simulink model "Problem_9"  (R2020a)
settings: Solver=VariableStepAuto  StartTime=0.0  StopTime=10.0  RelTol=1e-3
settings Model: Creator=user  LastModifiedBy=user

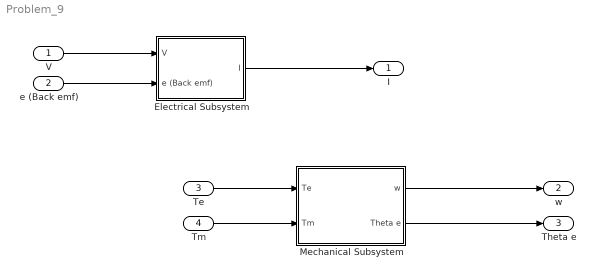
== system Problem_9 ==
  V : Inport
  e (Back emf) : Inport  Port=2
  Te : Inport  Port=3
  Tm : Inport  Port=4
  Electrical Subsystem : Subsystem
  Mechanical Subsystem : Subsystem
  I : Outport
  w : Outport  Port=2
  Theta e : Outport  Port=3
  wires:
  V/1 -> Electrical Subsystem/1(V)
  e (Back emf)/1 -> Electrical Subsystem/2(e (Back emf))
  Electrical Subsystem/1(I) -> I/1
  Te/1 -> Mechanical Subsystem/1(Te)
  Tm/1 -> Mechanical Subsystem/2(Tm)
  Mechanical Subsystem/1(w) -> w/1
  Mechanical Subsystem/2(Theta e) -> Theta e/1

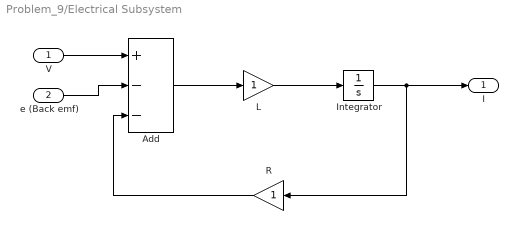
== system Problem_9/Electrical Subsystem ==
  V : Inport
  e (Back emf) : Inport  Port=2
  Add : Sum  Inputs=+--
  Integrator : Integrator
  L : Gain
  R : Gain
  I : Outport
  wires:
  Integrator/1 -> I/1, R/1
  Add/1 -> L/1
  R/1 -> Add/3
  e (Back emf)/1 -> Add/2
  L/1 -> Integrator/1
  V/1 -> Add/1

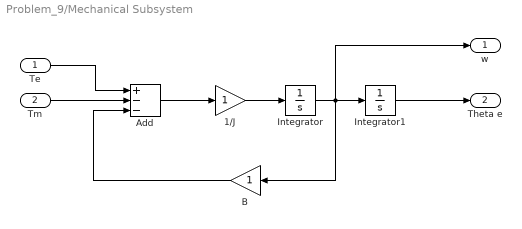
== system Problem_9/Mechanical Subsystem ==
  Te : Inport
  Tm : Inport  Port=2
  1/J : Gain
  Add : Sum  Inputs=+--
  B : Gain
  Integrator : Integrator
  Integrator1 : Integrator
  w : Outport
  Theta e : Outport  Port=2
  wires:
  Integrator1/1 -> Theta e/1
  Integrator/1 -> w/1, B/1, Integrator1/1
  Tm/1 -> Add/2
  Add/1 -> 1/J/1
  Te/1 -> Add/1
  1/J/1 -> Integrator/1
  B/1 -> Add/3
